simulink model "project_simulink"  (R2024a)
settings: Solver=VariableStepAuto  StartTime=0.0  StopTime=100  RelTol=1e-3
values from neighbouring files (symbols this model uses):
  b = 9.144    [aircraft_6dof.m]
  c = 3.45    [aircraft_6dof.m]
  delta_lef = 0    [aircraft_6dof.m]
  delta_r = 0    [aircraft_6dof.m]
  delta_sb = 0    [aircraft_6dof.m]
  f16_database =     [F16_LookupTables.mat]
  mass = 9300    [aircraft_6dof.m]
  S = 27.88    [aircraft_6dof.m]
  V_c = [153]    [aircraft_6dof.m]
libraries: aerolibconvert2 x5, shared6dof x1, aerolibatmos2 x1, aerolibasang x1
(part 2 of 2)

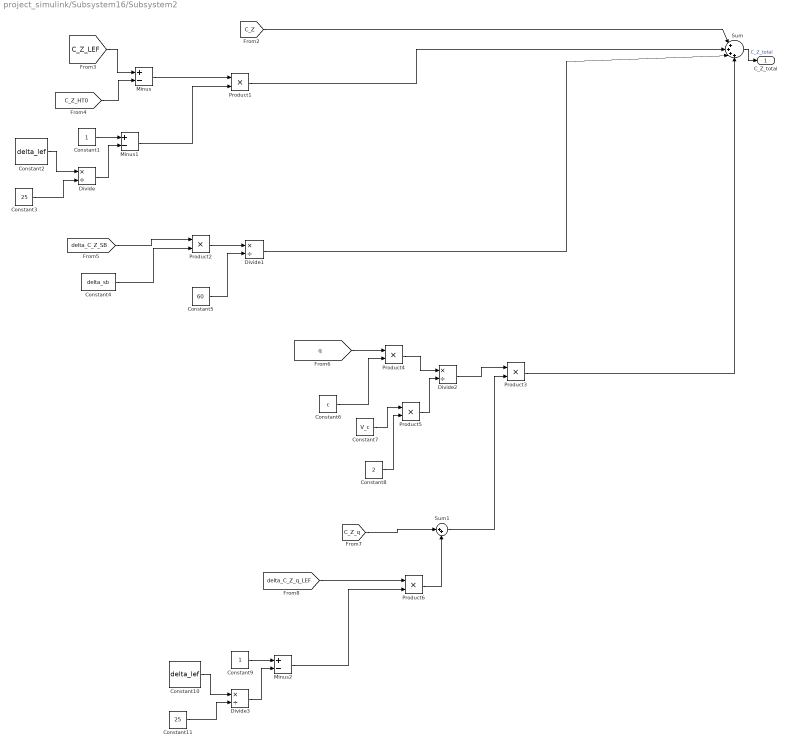
== system project_simulink/Subsystem16/Subsystem2 ==
  Constant1 : Constant
  Constant10 : Constant  Value=delta_lef
  Constant11 : Constant  Value=25
  Constant2 : Constant  Value=delta_lef
  Constant3 : Constant  Value=25
  Constant4 : Constant  Value=delta_sb
  Constant5 : Constant  Value=60
  Constant6 : Constant  Value=c
  Constant7 : Constant  Value=V_c
  Constant8 : Constant  Value=2
  Constant9 : Constant
  Divide{,1..3} (4 alike) : Product  Inputs=*/
  Minus : Sum  Inputs=+-
  Minus1 : Sum  Inputs=+-
  Minus2 : Sum  Inputs=+-
  Product{1..6} (6 alike) : Product
  Sum : Sum  Inputs=|++++
  Sum1 : Sum  Inputs=|++
  C_Z_total : Outport
  wires:
  Constant3/1 -> Divide/2
  Divide3/1 -> Minus2/2
  Constant2/1 -> Divide/1
  Constant5/1 -> Divide1/2
  [C_Z] -> Sum/1
  Divide/1 -> Minus1/2
  Divide2/1 -> Product3/1
  Product2/1 -> Divide1/1
  [q] -> Product4/1
  Product6/1 -> Sum1/2
  [delta_C_Z_SB] -> Product2/1
  Product3/1 -> Sum/4
  Constant7/1 -> Product5/1
  [C_Z_LEF] -> Minus/1
  [C_Z_q] -> Sum1/1
  Constant10/1 -> Divide3/1
  Constant8/1 -> Product5/2
  Minus2/1 -> Product6/2
  Sum1/1 -> Product3/2
  Divide1/1 -> Sum/3
  Constant11/1 -> Divide3/2
  Constant6/1 -> Product4/2
  Constant4/1 -> Product2/2
  Product1/1 -> Sum/2
  Minus/1 -> Product1/1
  [delta_C_Z_q_LEF] -> Product6/1
  Product5/1 -> Divide2/2
  Product4/1 -> Divide2/1
  Constant9/1 -> Minus2/1
  [C_Z_HT0] -> Minus/2
  Minus1/1 -> Product1/2
  Constant1/1 -> Minus1/1
  Sum/1 -> C_Z_total/1  "C_Z_total"

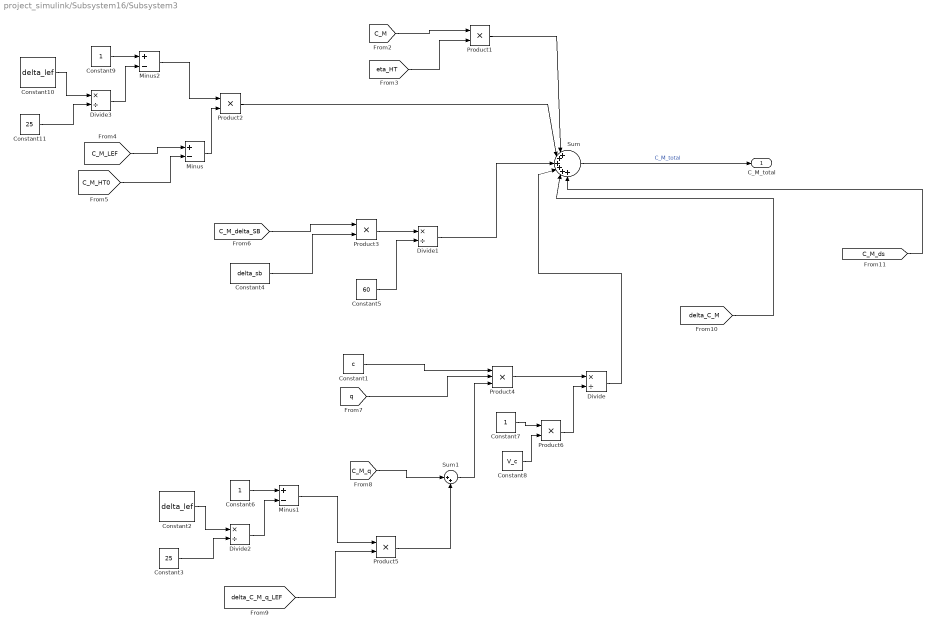
== system project_simulink/Subsystem16/Subsystem3 ==
  Constant1 : Constant  Value=c
  Constant10 : Constant  Value=delta_lef
  Constant11 : Constant  Value=25
  Constant2 : Constant  Value=delta_lef
  Constant3 : Constant  Value=25
  Constant4 : Constant  Value=delta_sb
  Constant5 : Constant  Value=60
  Constant6 : Constant
  Constant7 : Constant
  Constant8 : Constant  Value=V_c
  Constant9 : Constant
  Divide{,1..3} (4 alike) : Product  Inputs=*/
  Minus : Sum  Inputs=+-
  Minus1 : Sum  Inputs=+-
  Minus2 : Sum  Inputs=+-
  Product{1..3,5..6} (5 alike) : Product
  Product4 : Product  Inputs=3
  Sum : Sum  Inputs=|++++++
  Sum1 : Sum  Inputs=|++
  C_M_total : Outport
  wires:
  Divide3/1 -> Minus2/2
  Product4/1 -> Divide/1
  Product2/1 -> Sum/2
  Minus2/1 -> Product2/1
  Constant1/1 -> Product4/1
  Constant3/1 -> Divide2/2
  [eta_HT] -> Product1/2
  Divide1/1 -> Sum/3
  Constant4/1 -> Product3/2
  Constant11/1 -> Divide3/2
  [C_M] -> Product1/1
  [C_M_delta_SB] -> Product3/1
  Constant9/1 -> Minus2/1
  Constant10/1 -> Divide3/1
  [q] -> Product4/2
  [C_M_q] -> Sum1/1
  Constant8/1 -> Product6/2
  Product6/1 -> Divide/2
  Minus/1 -> Product2/2
  Sum1/1 -> Product4/3
  [delta_C_M_q_LEF] -> Product5/2
  Product1/1 -> Sum/1
  Divide/1 -> Sum/4
  Minus1/1 -> Product5/1
  Constant7/1 -> Product6/1
  [C_M_HT0] -> Minus/2
  Product3/1 -> Divide1/1
  Constant5/1 -> Divide1/2
  Product5/1 -> Sum1/2
  Constant2/1 -> Divide2/1
  Divide2/1 -> Minus1/2
  Constant6/1 -> Minus1/1
  Sum/1 -> C_M_total/1  "C_M_total"
  [C_M_ds] -> Sum/6
  [C_M_LEF] -> Minus/1
  [delta_C_M] -> Sum/5

== system project_simulink/Subsystem20/Subsystem16 ==
  Interpolation Using Prelookup1 : Interpolation_n-D  Table=f16_database.Engine.f16_EngineData.data.Thrust_lbs.idle  InternalRulePriority=Speed
  Length Conversion : aerolibconvert2/Length Conversion  IU=m  OU=ft
  Prelookup1 : PreLookup  BreakpointsData=f16_database.Engine.f16_EngineData.BP.idle.alt_ft  ExtrapMethod=Linear
  Prelookup3 : PreLookup  BreakpointsData=f16_database.Engine.f16_EngineData.BP.idle.mach  ExtrapMethod=Linear
  T_idle_N : Outport
  wires:
  Prelookup1/1 -> Interpolation Using Prelookup1/3
  Prelookup1/2 -> Interpolation Using Prelookup1/4
  Interpolation Using Prelookup1/1 -> T_idle_N/1  "T_idle_lbs"
  Length Conversion/1 -> Prelookup1/1  "altitude_ft"
  Prelookup3/1 -> Interpolation Using Prelookup1/1
  [Mach] -> Prelookup3/1  "mach"
  Prelookup3/2 -> Interpolation Using Prelookup1/2
  [h] -> Length Conversion/1

== system project_simulink/Subsystem20/Subsystem17 ==
  Interpolation Using Prelookup1 : Interpolation_n-D  Table=f16_database.Engine.f16_EngineData.data.Thrust_lbs.mil  InternalRulePriority=Speed
  Length Conversion : aerolibconvert2/Length Conversion  IU=m  OU=ft
  Prelookup1 : PreLookup  BreakpointsData=f16_database.Engine.f16_EngineData.BP.mil.alt_ft  ExtrapMethod=Linear
  Prelookup3 : PreLookup  BreakpointsData=f16_database.Engine.f16_EngineData.BP.mil.mach  ExtrapMethod=Linear
  T_mil_N : Outport
  wires:
  Prelookup3/1 -> Interpolation Using Prelookup1/1
  Prelookup1/1 -> Interpolation Using Prelookup1/3
  Length Conversion/1 -> Prelookup1/1  "altitude_ft"
  Prelookup3/2 -> Interpolation Using Prelookup1/2
  Prelookup1/2 -> Interpolation Using Prelookup1/4
  [Mach] -> Prelookup3/1  "mach"
  Interpolation Using Prelookup1/1 -> T_mil_N/1  "T_mil_N"
  [h] -> Length Conversion/1

== system project_simulink/Subsystem20/Subsystem19 ==
  Interpolation Using Prelookup2 : Interpolation_n-D  Table=f16_database.Engine.f16_EngineData.data.Thrust_lbs.max  InternalRulePriority=Speed
  Length Conversion : aerolibconvert2/Length Conversion  IU=m  OU=ft
  Prelookup2 : PreLookup  BreakpointsData=f16_database.Engine.f16_EngineData.BP.max.alt_ft  ExtrapMethod=Linear
  Prelookup4 : PreLookup  BreakpointsData=f16_database.Engine.f16_EngineData.BP.max.mach  ExtrapMethod=Linear
  T_max_N : Outport
  wires:
  Prelookup4/2 -> Interpolation Using Prelookup2/2
  Interpolation Using Prelookup2/1 -> T_max_N/1  "T_max_lbs"
  Prelookup2/2 -> Interpolation Using Prelookup2/4
  Prelookup2/1 -> Interpolation Using Prelookup2/3
  [Mach] -> Prelookup4/1  "mach"
  Length Conversion/1 -> Prelookup2/1  "altitude_ft"
  Prelookup4/1 -> Interpolation Using Prelookup2/1
  [h] -> Length Conversion/1

== system project_simulink/Subsystem21/Subsystem1 ==
  Interpolation Using Prelookup1 : Interpolation_n-D  Table=f16_database.f16_AerodynamicData.data.Cl.Clda20  InternalRulePriority=Speed
  Prelookup1 : PreLookup  BreakpointsData=f16_database.f16_AerodynamicData.BP.Cl.Clda20.beta  ExtrapMethod=Linear
  Prelookup3 : PreLookup  BreakpointsData=f16_database.f16_AerodynamicData.BP.Cl.Clda20.alpha  ExtrapMethod=Linear
  C_L_delta_a : Outport
  wires:
  Prelookup3/2 -> Interpolation Using Prelookup1/2
  [alpha] -> Prelookup3/1  "alpha"
  Prelookup3/1 -> Interpolation Using Prelookup1/1
  Interpolation Using Prelookup1/1 -> C_L_delta_a/1  "C_L_delta_a"
  Prelookup1/1 -> Interpolation Using Prelookup1/3
  Prelookup1/2 -> Interpolation Using Prelookup1/4
  [beta] -> Prelookup1/1  "beta"

== system project_simulink/Subsystem21/Subsystem13 ==
  Interpolation Using Prelookup1 : Interpolation_n-D  NumberOfTableDimensions=3  Table=f16_database.f16_AerodynamicData.data.Cl.Cl  InternalRulePriority=Speed
      settings: InputPortMap=u0,u1,u2,u3,u4,u5
  Prelookup3 : PreLookup  BreakpointsData=f16_database.f16_AerodynamicData.BP.Cl.Cl.alpha  ExtrapMethod=Linear
  Prelookup4 : PreLookup  BreakpointsData=f16_database.f16_AerodynamicData.BP.Cl.Cl.beta  ExtrapMethod=Linear
  Prelookup5 : PreLookup  BreakpointsData=f16_database.f16_AerodynamicData.BP.Cl.Cl.dHT  ExtrapMethod=Linear
  C_L : Outport
  wires:
  Prelookup4/1 -> Interpolation Using Prelookup1/3
  [alpha] -> Prelookup3/1  "alpha"
  Prelookup5/1 -> Interpolation Using Prelookup1/5
  [alpha] -> Prelookup4/1  "beta"
  Prelookup3/1 -> Interpolation Using Prelookup1/1
  [delta_e] -> Prelookup5/1  "dHT"
  Prelookup5/2 -> Interpolation Using Prelookup1/6
  Prelookup3/2 -> Interpolation Using Prelookup1/2
  Prelookup4/2 -> Interpolation Using Prelookup1/4
  Interpolation Using Prelookup1/1 -> C_L/1  "C_L"

== system project_simulink/Subsystem21/Subsystem14 ==
  Constant5 : Constant  Value=0
  Interpolation Using Prelookup1 : Interpolation_n-D  NumberOfTableDimensions=3  Table=f16_database.f16_AerodynamicData.data.Cl.Cl  InternalRulePriority=Speed
      settings: InputPortMap=u0,u1,u2,u3,u4,u5
  Prelookup3 : PreLookup  BreakpointsData=f16_database.f16_AerodynamicData.BP.Cl.Cl.alpha  ExtrapMethod=Linear
  Prelookup4 : PreLookup  BreakpointsData=f16_database.f16_AerodynamicData.BP.Cl.Cl.beta  ExtrapMethod=Linear
  Prelookup5 : PreLookup  BreakpointsData=f16_database.f16_AerodynamicData.BP.Cl.Cl.dHT  ExtrapMethod=Linear
  C_L_HT0 : Outport
  wires:
  Prelookup3/1 -> Interpolation Using Prelookup1/1
  Prelookup4/1 -> Interpolation Using Prelookup1/3
  [beta] -> Prelookup4/1  "beta"
  Prelookup3/2 -> Interpolation Using Prelookup1/2
  Prelookup5/1 -> Interpolation Using Prelookup1/5
  [alpha] -> Prelookup3/1  "alpha"
  Constant5/1 -> Prelookup5/1  "dHT"
  Prelookup4/2 -> Interpolation Using Prelookup1/4
  Prelookup5/2 -> Interpolation Using Prelookup1/6
  Interpolation Using Prelookup1/1 -> C_L_HT0/1  "C_L_HT0"

== system project_simulink/Subsystem21/Subsystem16 ==
  Interpolation Using Prelookup1 : Interpolation_n-D  NumberOfTableDimensions=1  Table=f16_database.f16_AerodynamicData.data.Cl.Clr  InternalRulePriority=Speed
      settings: InputPortMap=u0,u1
  Prelookup3 : PreLookup  BreakpointsData=f16_database.f16_AerodynamicData.BP.Cl.Clr.alpha  ExtrapMethod=Linear
  C_L_r : Outport
  wires:
  Interpolation Using Prelookup1/1 -> C_L_r/1  "C_L_r"
  [alpha] -> Prelookup3/1  "alpha"
  Prelookup3/1 -> Interpolation Using Prelookup1/1
  Prelookup3/2 -> Interpolation Using Prelookup1/2

== system project_simulink/Subsystem21/Subsystem17 ==
  Interpolation Using Prelookup1 : Interpolation_n-D  NumberOfTableDimensions=1  Table=f16_database.f16_AerodynamicData.data.Cl.deltaClrlef  InternalRulePriority=Speed
      settings: InputPortMap=u0,u1
  Prelookup3 : PreLookup  BreakpointsData=f16_database.f16_AerodynamicData.BP.Cl.deltaClrlef.alpha  ExtrapMethod=Linear
  delta_C_L_r_LEF : Outport
  wires:
  Prelookup3/1 -> Interpolation Using Prelookup1/1
  Prelookup3/2 -> Interpolation Using Prelookup1/2
  [alpha] -> Prelookup3/1  "alpha"
  Interpolation Using Prelookup1/1 -> delta_C_L_r_LEF/1  "delta_C_L_r_LEF"

== system project_simulink/Subsystem21/Subsystem18 ==
  Interpolation Using Prelookup1 : Interpolation_n-D  NumberOfTableDimensions=1  Table=f16_database.f16_AerodynamicData.data.Cl.Clp  InternalRulePriority=Speed
      settings: InputPortMap=u0,u1
  Prelookup3 : PreLookup  BreakpointsData=f16_database.f16_AerodynamicData.BP.Cl.Clp.alpha  ExtrapMethod=Linear
  C_L_p : Outport
  wires:
  [alpha] -> Prelookup3/1  "alpha"
  Prelookup3/1 -> Interpolation Using Prelookup1/1
  Prelookup3/2 -> Interpolation Using Prelookup1/2
  Interpolation Using Prelookup1/1 -> C_L_p/1  "C_L_p"

== system project_simulink/Subsystem21/Subsystem19 ==
  Interpolation Using Prelookup1 : Interpolation_n-D  NumberOfTableDimensions=1  Table=f16_database.f16_AerodynamicData.data.Cl.deltaClplef  InternalRulePriority=Speed
      settings: InputPortMap=u0,u1
  Prelookup3 : PreLookup  BreakpointsData=f16_database.f16_AerodynamicData.BP.Cl.deltaClplef.alpha  ExtrapMethod=Linear
  delta_C_L_p_LEF : Outport
  wires:
  [alpha] -> Prelookup3/1  "alpha"
  Interpolation Using Prelookup1/1 -> delta_C_L_p_LEF/1  "delta_C_L_p_LEF"
  Prelookup3/1 -> Interpolation Using Prelookup1/1
  Prelookup3/2 -> Interpolation Using Prelookup1/2

== system project_simulink/Subsystem21/Subsystem2 ==
  Interpolation Using Prelookup1 : Interpolation_n-D  Table=f16_database.f16_AerodynamicData.data.Cl.Cldr30  InternalRulePriority=Speed
  Prelookup1 : PreLookup  BreakpointsData=f16_database.f16_AerodynamicData.BP.Cl.Cldr30.beta  ExtrapMethod=Linear
  Prelookup3 : PreLookup  BreakpointsData=f16_database.f16_AerodynamicData.BP.Cl.Cldr30.alpha  ExtrapMethod=Linear
  C_L_delta_r : Outport
  wires:
  Prelookup3/2 -> Interpolation Using Prelookup1/2
  [alpha] -> Prelookup3/1  "alpha"
  Prelookup3/1 -> Interpolation Using Prelookup1/1
  Interpolation Using Prelookup1/1 -> C_L_delta_r/1  "C_L_delta_r"
  Prelookup1/1 -> Interpolation Using Prelookup1/3
  Prelookup1/2 -> Interpolation Using Prelookup1/4
  [beta] -> Prelookup1/1  "beta"

== system project_simulink/Subsystem21/Subsystem20 ==
  Interpolation Using Prelookup1 : Interpolation_n-D  NumberOfTableDimensions=1  Table=f16_database.f16_AerodynamicData.data.Cl.deltaClBeta  InternalRulePriority=Speed
      settings: InputPortMap=u0,u1
  Prelookup3 : PreLookup  BreakpointsData=f16_database.f16_AerodynamicData.BP.Cl.deltaClBeta.alpha  ExtrapMethod=Linear
  delta_C_L_beta : Outport
  wires:
  Prelookup3/2 -> Interpolation Using Prelookup1/2
  [alpha] -> Prelookup3/1  "alpha"
  Prelookup3/1 -> Interpolation Using Prelookup1/1
  Interpolation Using Prelookup1/1 -> delta_C_L_beta/1  "delta_C_L_beta"

== system project_simulink/Subsystem21/Subsystem3 ==
  Interpolation Using Prelookup1 : Interpolation_n-D  Table=f16_database.f16_AerodynamicData.data.Cl.Clda20lef  InternalRulePriority=Speed
  Prelookup1 : PreLookup  BreakpointsData=f16_database.f16_AerodynamicData.BP.Cl.Clda20lef.beta  ExtrapMethod=Linear
  Prelookup3 : PreLookup  BreakpointsData=f16_database.f16_AerodynamicData.BP.Cl.Clda20lef.alpha  ExtrapMethod=Linear
  C_L_delta_a_LEF : Outport
  wires:
  Prelookup3/2 -> Interpolation Using Prelookup1/2
  [alpha] -> Prelookup3/1  "alpha"
  Prelookup3/1 -> Interpolation Using Prelookup1/1
  Interpolation Using Prelookup1/1 -> C_L_delta_a_LEF/1  "C_L_delta_a_LEF"
  Prelookup1/1 -> Interpolation Using Prelookup1/3
  Prelookup1/2 -> Interpolation Using Prelookup1/4
  [beta] -> Prelookup1/1  "beta"

== system project_simulink/Subsystem21/Subsystem4 ==
  Interpolation Using Prelookup2 : Interpolation_n-D  Table=f16_database.f16_AerodynamicData.data.Cl.Cllef  InternalRulePriority=Speed
  Prelookup2 : PreLookup  BreakpointsData=f16_database.f16_AerodynamicData.BP.Cl.Cllef.alpha  ExtrapMethod=Linear
  Prelookup4 : PreLookup  BreakpointsData=f16_database.f16_AerodynamicData.BP.Cl.Cllef.beta  ExtrapMethod=Linear
  C_L_LEF : Outport
  wires:
  [alpha] -> Prelookup2/1  "alpha"
  Prelookup4/2 -> Interpolation Using Prelookup2/4
  Interpolation Using Prelookup2/1 -> C_L_LEF/1  "C_L_LEF"
  Prelookup4/1 -> Interpolation Using Prelookup2/3
  Prelookup2/2 -> Interpolation Using Prelookup2/2
  Prelookup2/1 -> Interpolation Using Prelookup2/1
  [beta] -> Prelookup4/1  "beta"

== system project_simulink/Subsystem6/Subsystem ==
  Interpolation Using Prelookup4 : Interpolation_n-D  NumberOfTableDimensions=3  Table=f16_database.f16_AerodynamicData.data.CZ.CZ  InternalRulePriority=Speed
      settings: InputPortMap=u0,u1,u2,u3,u4,u5
  Prelookup1 : PreLookup  BreakpointsData=f16_database.f16_AerodynamicData.BP.CZ.CZ.dHT  ExtrapMethod=Linear
  Prelookup8 : PreLookup  BreakpointsData=f16_database.f16_AerodynamicData.BP.CZ.CZ.alpha  ExtrapMethod=Linear
  Prelookup9 : PreLookup  BreakpointsData=f16_database.f16_AerodynamicData.BP.CZ.CZ.beta  ExtrapMethod=Linear
  C_Z : Outport
  wires:
  Prelookup8/2 -> Interpolation Using Prelookup4/2
  Prelookup8/1 -> Interpolation Using Prelookup4/1
  Prelookup1/2 -> Interpolation Using Prelookup4/6
  [beta] -> Prelookup9/1
  Prelookup1/1 -> Interpolation Using Prelookup4/5
  [delta_e] -> Prelookup1/1
  Prelookup9/2 -> Interpolation Using Prelookup4/4
  [alpha] -> Prelookup8/1
  Prelookup9/1 -> Interpolation Using Prelookup4/3
  Interpolation Using Prelookup4/1 -> C_Z/1  "C_Z"

== system project_simulink/Subsystem6/Subsystem1 ==
  Constant6 : Constant  Value=0
  Interpolation Using Prelookup3 : Interpolation_n-D  NumberOfTableDimensions=3  Table=f16_database.f16_AerodynamicData.data.CZ.CZ  InternalRulePriority=Speed
      settings: InputPortMap=u0,u1,u2,u3,u4,u5
  Prelookup10 : PreLookup  BreakpointsData=f16_database.f16_AerodynamicData.BP.CZ.CZ.beta  ExtrapMethod=Linear
  Prelookup6 : PreLookup  BreakpointsData=f16_database.f16_AerodynamicData.BP.CZ.CZ.dHT  ExtrapMethod=Linear
  Prelookup7 : PreLookup  BreakpointsData=f16_database.f16_AerodynamicData.BP.CZ.CZ.alpha  ExtrapMethod=Linear
  C_Z_HT0 : Outport
  wires:
  Prelookup6/2 -> Interpolation Using Prelookup3/6
  [beta] -> Prelookup10/1
  Prelookup7/1 -> Interpolation Using Prelookup3/1
  Interpolation Using Prelookup3/1 -> C_Z_HT0/1  "C_Z_HT0"
  Prelookup10/1 -> Interpolation Using Prelookup3/3
  Constant6/1 -> Prelookup6/1
  Prelookup7/2 -> Interpolation Using Prelookup3/2
  [alpha] -> Prelookup7/1
  Prelookup6/1 -> Interpolation Using Prelookup3/5
  Prelookup10/2 -> Interpolation Using Prelookup3/4

== system project_simulink/Subsystem6/Subsystem2 ==
  Interpolation Using Prelookup1 : Interpolation_n-D  Table=f16_database.f16_AerodynamicData.data.CZ.CZlef  InternalRulePriority=Speed
  Prelookup3 : PreLookup  BreakpointsData=f16_database.f16_AerodynamicData.BP.CZ.CZlef.alpha  ExtrapMethod=Linear
  Prelookup4 : PreLookup  BreakpointsData=f16_database.f16_AerodynamicData.BP.CZ.CZlef.beta  ExtrapMethod=Linear
  C_Z_LEF : Outport
  wires:
  Interpolation Using Prelookup1/1 -> C_Z_LEF/1  "C_Z_LEF"
  Prelookup4/2 -> Interpolation Using Prelookup1/4
  [alpha] -> Prelookup3/1
  Prelookup3/1 -> Interpolation Using Prelookup1/1
  [beta] -> Prelookup4/1
  Prelookup4/1 -> Interpolation Using Prelookup1/3
  Prelookup3/2 -> Interpolation Using Prelookup1/2

== system project_simulink/Subsystem6/Subsystem3 ==
  Interpolation Using Prelookup2 : Interpolation_n-D  NumberOfTableDimensions=1  Table=f16_database.f16_AerodynamicData.data.CZ.deltaCZSB  InternalRulePriority=Speed
      settings: InputPortMap=u0,u1
  Prelookup2 : PreLookup  BreakpointsData=f16_database.f16_AerodynamicData.BP.CZ.deltaCZSB.alpha  ExtrapMethod=Linear
  delta_C_Z_SB : Outport
  wires:
  Interpolation Using Prelookup2/1 -> delta_C_Z_SB/1  "delta_C_Z_SB"
  Prelookup2/1 -> Interpolation Using Prelookup2/1
  Prelookup2/2 -> Interpolation Using Prelookup2/2
  [alpha] -> Prelookup2/1

== system project_simulink/Subsystem6/Subsystem4 ==
  Interpolation Using Prelookup5 : Interpolation_n-D  NumberOfTableDimensions=1  Table=f16_database.f16_AerodynamicData.data.CZ.CZq  InternalRulePriority=Speed
      settings: InputPortMap=u0,u1
  Prelookup5 : PreLookup  BreakpointsData=f16_database.f16_AerodynamicData.BP.CZ.CZq.alpha  ExtrapMethod=Linear
  C_Z_q : Outport
  wires:
  Prelookup5/2 -> Interpolation Using Prelookup5/2
  Interpolation Using Prelookup5/1 -> C_Z_q/1  "C_Z_q"
  Prelookup5/1 -> Interpolation Using Prelookup5/1
  [alpha] -> Prelookup5/1

== system project_simulink/Subsystem6/Subsystem5 ==
  Interpolation Using Prelookup6 : Interpolation_n-D  NumberOfTableDimensions=1  Table=f16_database.f16_AerodynamicData.data.CZ.deltaCZqlef  InternalRulePriority=Speed
      settings: InputPortMap=u0,u1
  Prelookup11 : PreLookup  BreakpointsData=f16_database.f16_AerodynamicData.BP.CZ.deltaCZqlef.alpha  ExtrapMethod=Linear
  delta_C_Z_q_LEF : Outport
  wires:
  Prelookup11/2 -> Interpolation Using Prelookup6/2
  [alpha] -> Prelookup11/1
  Interpolation Using Prelookup6/1 -> delta_C_Z_q_LEF/1  "delta_C_Z_q_LEF"
  Prelookup11/1 -> Interpolation Using Prelookup6/1

== system project_simulink/Subsystem7/Subsystem ==
  Interpolation Using Prelookup : Interpolation_n-D  NumberOfTableDimensions=3  Table=f16_database.f16_AerodynamicData.data.CX.CX  InternalRulePriority=Speed
      settings: InputPortMap=u0,u1,u2,u3,u4,u5
  Prelookup : PreLookup  BreakpointsData=f16_database.f16_AerodynamicData.BP.CX.CX.alpha  ExtrapMethod=Linear
  Prelookup1 : PreLookup  BreakpointsData=f16_database.f16_AerodynamicData.BP.CX.CX.beta  ExtrapMethod=Linear
  Prelookup2 : PreLookup  BreakpointsData=f16_database.f16_AerodynamicData.BP.CX.CX.dHT  ExtrapMethod=Linear
  C_X : Outport
  wires:
  Interpolation Using Prelookup/1 -> C_X/1  "C_X"
  Prelookup1/1 -> Interpolation Using Prelookup/3
  Prelookup2/2 -> Interpolation Using Prelookup/6
  [beta] -> Prelookup1/1  "beta"
  [alpha] -> Prelookup/1  "alpha"
  [delta_e] -> Prelookup2/1  "dHT"
  Prelookup/2 -> Interpolation Using Prelookup/2
  Prelookup1/2 -> Interpolation Using Prelookup/4
  Prelookup/1 -> Interpolation Using Prelookup/1
  Prelookup2/1 -> Interpolation Using Prelookup/5

== system project_simulink/Subsystem7/Subsystem1 ==
  Constant5 : Constant  Value=0
  Interpolation Using Prelookup1 : Interpolation_n-D  NumberOfTableDimensions=3  Table=f16_database.f16_AerodynamicData.data.CX.CX  InternalRulePriority=Speed
      settings: InputPortMap=u0,u1,u2,u3,u4,u5
  Prelookup3 : PreLookup  BreakpointsData=f16_database.f16_AerodynamicData.BP.CX.CX.alpha  ExtrapMethod=Linear
  Prelookup4 : PreLookup  BreakpointsData=f16_database.f16_AerodynamicData.BP.CX.CX.beta  ExtrapMethod=Linear
  Prelookup5 : PreLookup  BreakpointsData=f16_database.f16_AerodynamicData.BP.CX.CX.dHT  ExtrapMethod=Linear
  C_X_HT0 : Outport
  wires:
  Prelookup5/1 -> Interpolation Using Prelookup1/5
  [beta] -> Prelookup4/1  "beta"
  Prelookup3/2 -> Interpolation Using Prelookup1/2
  Prelookup4/2 -> Interpolation Using Prelookup1/4
  Prelookup4/1 -> Interpolation Using Prelookup1/3
  Prelookup3/1 -> Interpolation Using Prelookup1/1
  Constant5/1 -> Prelookup5/1  "dHT"
  Prelookup5/2 -> Interpolation Using Prelookup1/6
  [alpha] -> Prelookup3/1  "alpha"
  Interpolation Using Prelookup1/1 -> C_X_HT0/1  "C_X_HT0"

== system project_simulink/Subsystem7/Subsystem2 ==
  Interpolation Using Prelookup2 : Interpolation_n-D  Table=f16_database.f16_AerodynamicData.data.CX.CXlef  InternalRulePriority=Speed
  Prelookup6 : PreLookup  BreakpointsData=f16_database.f16_AerodynamicData.BP.CX.CXlef.alpha  ExtrapMethod=Linear
  Prelookup7 : PreLookup  BreakpointsData=f16_database.f16_AerodynamicData.BP.CX.CXlef.beta  ExtrapMethod=Linear
  C_X_LEF : Outport
  wires:
  Prelookup7/2 -> Interpolation Using Prelookup2/4
  [beta] -> Prelookup7/1
  Interpolation Using Prelookup2/1 -> C_X_LEF/1  "C_X_LEF"
  Prelookup6/2 -> Interpolation Using Prelookup2/2
  Prelookup6/1 -> Interpolation Using Prelookup2/1
  [alpha] -> Prelookup6/1
  Prelookup7/1 -> Interpolation Using Prelookup2/3

== system project_simulink/Subsystem7/Subsystem3 ==
  Interpolation Using Prelookup3 : Interpolation_n-D  NumberOfTableDimensions=1  Table=f16_database.f16_AerodynamicData.data.CX.CXq  InternalRulePriority=Speed
      settings: InputPortMap=u0,u1
  Prelookup8 : PreLookup  BreakpointsData=f16_database.f16_AerodynamicData.BP.CX.CXq.alpha  ExtrapMethod=Linear
  C_X_q : Outport
  wires:
  Prelookup8/1 -> Interpolation Using Prelookup3/1
  [alpha] -> Prelookup8/1
  Prelookup8/2 -> Interpolation Using Prelookup3/2
  Interpolation Using Prelookup3/1 -> C_X_q/1  "C_X_q"

== system project_simulink/Subsystem7/Subsystem4 ==
  Interpolation Using Prelookup5 : Interpolation_n-D  NumberOfTableDimensions=1  Table=f16_database.f16_AerodynamicData.data.CX.deltaCXSB  InternalRulePriority=Speed
      settings: InputPortMap=u0,u1
  Prelookup10 : PreLookup  BreakpointsData=f16_database.f16_AerodynamicData.BP.CX.deltaCXSB.alpha  ExtrapMethod=Linear
  C_X_SB : Outport
  wires:
  Prelookup10/1 -> Interpolation Using Prelookup5/1
  [alpha] -> Prelookup10/1
  Prelookup10/2 -> Interpolation Using Prelookup5/2
  Interpolation Using Prelookup5/1 -> C_X_SB/1  "C_X_SB"

== system project_simulink/Subsystem7/Subsystem5 ==
  Interpolation Using Prelookup4 : Interpolation_n-D  NumberOfTableDimensions=1  Table=f16_database.f16_AerodynamicData.data.CX.deltaCXqlef  InternalRulePriority=Speed
      settings: InputPortMap=u0,u1
  Prelookup9 : PreLookup  BreakpointsData=f16_database.f16_AerodynamicData.BP.CX.deltaCXqlef.alpha  ExtrapMethod=Linear
  delta_C_X_qLEF : Outport
  wires:
  Prelookup9/1 -> Interpolation Using Prelookup4/1
  Interpolation Using Prelookup4/1 -> delta_C_X_qLEF/1  "delta_C_X_qLEF"
  Prelookup9/2 -> Interpolation Using Prelookup4/2
  [alpha] -> Prelookup9/1

== system project_simulink/Subsystem10/Subsystem4/Subsystem3 ==
  Interpolation Using Prelookup3 : Interpolation_n-D  Table=f16_database.f16_AerodynamicData.data.CY.CYda20lef  InternalRulePriority=Speed
  Prelookup6 : PreLookup  BreakpointsData=f16_database.f16_AerodynamicData.BP.CY.CYda20lef.alpha  ExtrapMethod=Linear
  Prelookup7 : PreLookup  BreakpointsData=f16_database.f16_AerodynamicData.BP.CY.CYda20lef.beta  ExtrapMethod=Linear
  C_Y_delta_a_LEF : Outport
  wires:
  [alpha] -> Prelookup6/1
  Prelookup7/2 -> Interpolation Using Prelookup3/4
  Interpolation Using Prelookup3/1 -> C_Y_delta_a_LEF/1  "C_Y_delta_a_LEF"
  Prelookup6/2 -> Interpolation Using Prelookup3/2
  Prelookup6/1 -> Interpolation Using Prelookup3/1
  [beta] -> Prelookup7/1
  Prelookup7/1 -> Interpolation Using Prelookup3/3

== system project_simulink/Subsystem16/Subsystem11/Subsystem4 ==
  Minus : Sum  Inputs=+-
  delta_C_N_LEF : Outport
  wires:
  [C_NHT0] -> Minus/2
  [C_N_LEF] -> Minus/1
  Minus/1 -> delta_C_N_LEF/1  "delta_C_N_LEF"

== system project_simulink/Subsystem16/Subsystem11/Subsystem5 ==
  Minus : Sum  Inputs=+-
  delta_C_N_delta_a : Outport
  wires:
  [C_NHT0] -> Minus/2
  [C_N_delta_a] -> Minus/1
  Minus/1 -> delta_C_N_delta_a/1  "delta_C_N_delta_a"

== system project_simulink/Subsystem16/Subsystem11/Subsystem8 ==
  Minus : Sum  Inputs=+--
  delta_C_N_delta_a_LEF : Outport
  wires:
  [C_N_delta_a_LEF] -> Minus/1
  [C_N_LEF] -> Minus/2
  [delta_C_N_delta_a] -> Minus/3
  Minus/1 -> delta_C_N_delta_a_LEF/1  "delta_C_N_delta_a_LEF"

== system project_simulink/Subsystem16/Subsystem11/Subsystem9 ==
  Minus : Sum  Inputs=+-
  delta_C_N_delta_r : Outport
  wires:
  [C_N_delta_r] -> Minus/1
  [C_NHT0] -> Minus/2
  Minus/1 -> delta_C_N_delta_r/1  "delta_C_N_delta_r"

== system project_simulink/Subsystem16/Subsystem18/Subsystem13 ==
  Minus : Sum  Inputs=+-
  delta_C_L_LEF : Outport
  wires:
  [C_L_HT0] -> Minus/2
  [C_L_LEF] -> Minus/1
  Minus/1 -> delta_C_L_LEF/1  "delta_C_L_LEF"

== system project_simulink/Subsystem16/Subsystem18/Subsystem14 ==
  Minus : Sum  Inputs=+-
  delta_C_L_delta_a : Outport
  wires:
  [C_L_HT0] -> Minus/2
  [C_L_delta_a] -> Minus/1
  Minus/1 -> delta_C_L_delta_a/1  "delta_C_L_delta_a"

== system project_simulink/Subsystem16/Subsystem18/Subsystem16 ==
  Minus : Sum  Inputs=+--
  delta_C_L_delta_a_LEF : Outport
  wires:
  [C_L_delta_a_LEF] -> Minus/1
  [C_L_LEF] -> Minus/2
  [delta_C_L_delta_a] -> Minus/3
  Minus/1 -> delta_C_L_delta_a_LEF/1  "delta_C_L_delta_a_LEF"

== system project_simulink/Subsystem16/Subsystem18/Subsystem17 ==
  Minus : Sum  Inputs=+-
  delta_C_L_delta_r : Outport
  wires:
  [C_L_delta_r] -> Minus/1
  [C_L_HT0] -> Minus/2
  Minus/1 -> delta_C_L_delta_r/1  "delta_C_L_delta_r"

== matlab function project_simulink/MATLAB Function ==
  data: T_idle input; T output; T_mil input; T_max input; Pc input
function T = thrustcal(T_idle, T_mil,T_max, Pc)

if Pc < 50
    T = T_idle + (T_mil-T_idle)*Pc/50;
    
else Pc >= 50
    T = T_mil + (T_max-T_mil)*(Pc-50)/50;
end

end
